simulink model "vehicle_simulation"  (R2015a)
settings: Solver=ode45  StartTime=0.0  StopTime=10.0  RelTol=1e-3
values from neighbouring files (symbols this model uses):
  ddr = zeros(size(x))    [signalgen.m]    (also in temp.m)
  phi = atan(dr)    [signalgen.m]    (also in temp.m)
  r = cumsum(dr)*dx    [signalgen.m]    (also in temp.m)
  x = xout.Data    [animation.m]    (also in signalgen.m = 0:dx:10; temp.m = 0:dx:10)
settings Model: Creator=tvincent  LastModifiedBy=tvincent

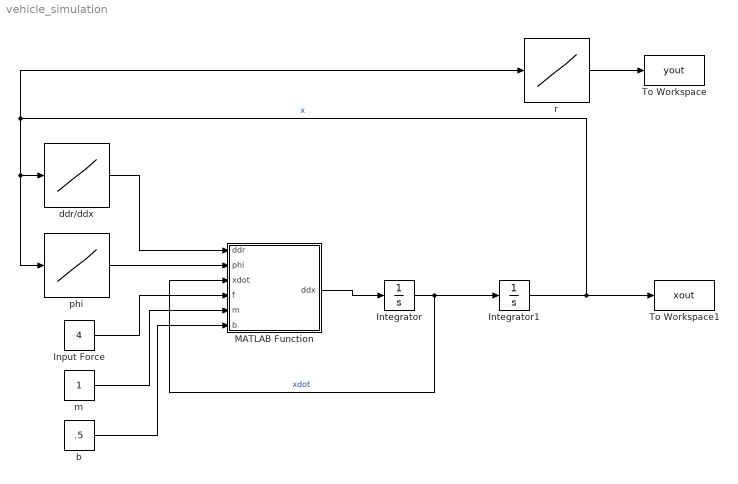
== system vehicle_simulation ==
  Input Force : Constant  Value=4
  Integrator : Integrator
  Integrator1 : Integrator
  MATLAB Function : MATLAB Function  TreatAsAtomicUnit=on
  To Workspace : ToWorkspace  VariableName=yout  SaveFormat=Timeseries  SampleTime=-1
  To Workspace1 : ToWorkspace  VariableName=xout  SaveFormat=Timeseries  SampleTime=-1
  b : Constant  Value=.5
  ddr/ddx : Lookup_n-D  NumberOfTableDimensions=1  BreakpointsForDimension1=x  Table=ddr  InternalRulePriority=Speed  RndMeth=Simplest  InputSameDT=on
  m : Constant
  phi : Lookup_n-D  NumberOfTableDimensions=1  BreakpointsForDimension1=x  Table=phi  InternalRulePriority=Speed  RndMeth=Simplest  InputSameDT=on
  r : Lookup_n-D  NumberOfTableDimensions=1  BreakpointsForDimension1=x  Table=r  InternalRulePriority=Speed  RndMeth=Simplest  InputSameDT=on
  wires:
  phi/1 -> MATLAB Function/2(phi)
  MATLAB Function/1(ddx) -> Integrator/1
  Integrator/1 -> MATLAB Function/3(xdot), Integrator1/1  "xdot"
  Integrator1/1 -> phi/1, ddr/ddx/1, r/1, To Workspace1/1  "x"
  ddr/ddx/1 -> MATLAB Function/1(ddr)
  Input Force/1 -> MATLAB Function/4(f)
  r/1 -> To Workspace/1
  b/1 -> MATLAB Function/6(b)
  m/1 -> MATLAB Function/5(m)

== matlab function vehicle_simulation/MATLAB Function ==
  data: ddr input; phi input; ddx output; xdot input; f input; m input; b input
function ddx = fcn(ddr,phi,xdot,f,m,b)
%#codegen
g=9.81;


ddx = cos(phi)*(-ddr*xdot^2*sin(phi) - g*sin(phi) + (1/m)*f - (b/cos(phi))*xdot);
